simulink model "APVWith3DSimulation"  (R2022b)
settings: Solver=ode23tb  StartTime=0.0  StopTime=inf  MaxStep=1e-2  MinStep=1e-3  RelTol=1e-2
PreLoadFcn:
  | helperSLCreateUtilityBus(1);
StopFcn:
  | clear helperSLVisualizePath;
values from neighbouring files (symbols this model uses):
  costmap = vehicleCostmap(costmapStruct.Costs,          'FreeThreshold',     costmapStruct.FreeThreshold,          'OccupiedThreshold', costmapStruct.OccupiedThreshold,          'MapLocation',       costmapStruct.MapExtent([1, 3]),          'CellSize',          costmapStruct.CellSize,          'CollisionChecker',  ccConfig)    [helperSLVisualizePath.m]
undefined symbols (not defined in the file or in its folder): centerToRear, routePlan, startPose
libraries: drivinglib x2, drivingvehiclecontroller x2, simulink x2, simulink_extras x2, sim3dlib x1, sim3dautolib x1, autolibshared x1
CloseFcn:
  | clear plannerConfigBus ...
  | speedConfigBus ...
  | vehicleInfoBus ...
  | startPose ...
  | costmap ...
  | routeData ...
  | routePlan;
settings Model: Creator=The MathWorks, Inc.  LastModifiedBy=The MathWorks, Inc.
settings SolverCC: MaxConsecutiveMinStep=2  ZeroCrossAlgorithm=Adaptive  AlgebraicLoopSolver=TrustRegion  DecoupledContinuousIntegration=on  MinimalZcImpactIntegration=on
settings DataIOCC: SaveOutput=off  SignalLogging=off  DSMLogging=off  SaveTime=off  ReturnWorkspaceOutputs=off
settings DebuggingCC: UnconnectedInputMsg=warning  UnconnectedOutputMsg=warning  UnconnectedLineMsg=warning  PregeneratedLibrarySubsystemCodeDiagnostic=none  SFMachineParentedDataDiag=warning  ArithmeticOperatorsInVariantConditions=warning
settings ModelReferenceCC: EnableRefExpFcnMdlSchedulingChecks=on
settings SFSimCC: SimUseLocalCustomCode=off
settings RTWCC: RTWUseLocalCustomCode=off  DLArmComputeVersion=19.05

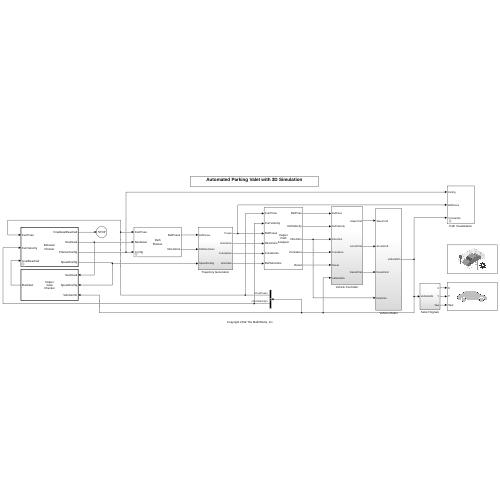
[thumbnail: Simulink's stored preview of the top-level diagram]
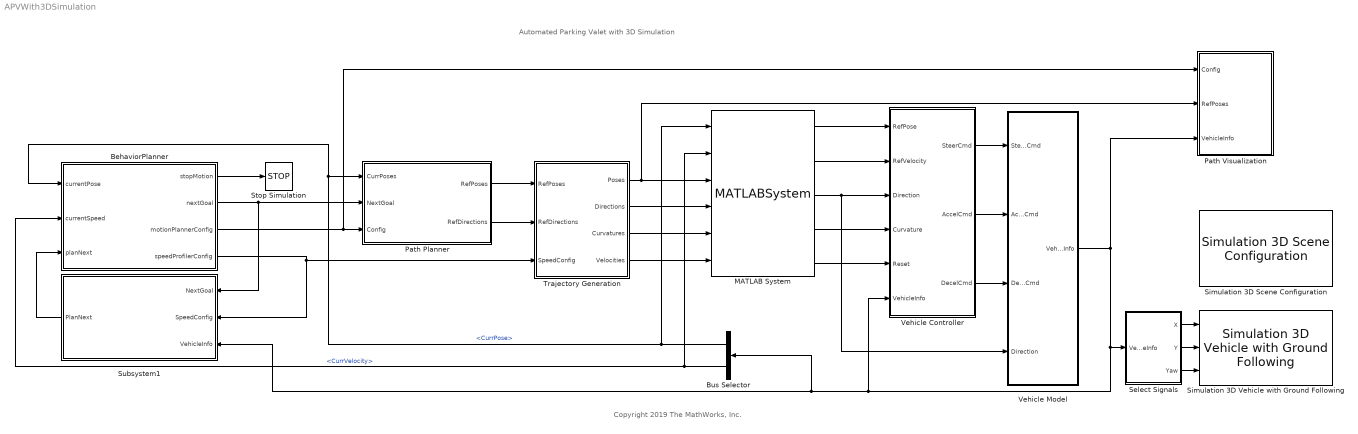
== system APVWith3DSimulation ==
  note: Copyright 2019 The MathWorks, Inc.
  note: Automated Parking Valet with 3D Simulation
  BehaviorPlanner : MATLAB Function  TreatAsAtomicUnit=on  mask{Costmap=costmap, RoutePlan=routePlan, StartSpeed=0}
      mask prompts: Costmap "Vehicle costmap:"; RoutePlan "Route plan:"; StartSpeed "Initial vehicle speed  [m/s]:"
      mask init:
      | validateattributes(Costmap, {'vehicleCostmap'}, {'scalar'});
      | validateattributes(RoutePlan, {'table'}, {'ncols', 3});
      | validateattributes(StartSpeed, {'double'}, {'scalar','nonnegative'})
      | 
      | routePlanStruct   = table2struct(RoutePlan);
      | startPose         = routePlanStruct(1).StartPose;
      | 
      | varagout          = helperSLCreateUtilityStruct(Costmap);
      | vehicleDimsStruct = varagout{1};
      | costmapStruct     = varagout{2};
  Bus Selector : BusSelector  OutputSignals=CurrPose,CurrVelocity
  MATLAB System : MATLABSystem  System=HelperPathAnalyzer  Wheelbase=2.6  HasResetOutput=on  SimulateUsing=Interpreted execution
      mask Type: HelperPathAnalyzer
      mask Display:
      | disp(['Helper' char(10) 'Path' char(10) 'Analyzer']);
      | port_label('input',1,'CurrPose');
      | port_label('input',2,'CurrVelocity');
      | port_label('input',3,'RefPoses');
      | port_label('input',4,'Directions');
      | port_label('input',5,'Curvatures');
      | port_label('input',6,'RefVelocities');
      | port_label('output',1,'RefPose');
      | port_label('output',2,'RefVelocity');
      | port_label('output',3,'Direction');
      | port_label('output',4,'Curvature');
      | port_label('output',5,'Reset');
  Path Planner : Subsystem  mask{Costmap=costmap, ParkCostmapSize=30}
      mask prompts: Costmap "Global vehicle costmap:"; ParkCostmapSize "Local vehicle costmap size (m):"
      mask init:
      | varagout = helperSLCreateUtilityStruct(Costmap);
      | vehicleDimsStruct = varagout{1};
      | costmapStruct     = varagout{2};
      mask DialogControl DescGroupVar Prompt: Path Planner Helper
      mask Display:
      | disp(['Path' char(10) 'Planner']);
      | port_label('input',1,'CurrPose');
      | port_label('input',2,'NextGoal');
      | port_label('input',3,'Config');
      | port_label('output',1,'RefPoses');
      | port_label('output',2,'Directions');
  Path Visualization : Subsystem  mask{Costmap=costmap, ParkCostmapSize=30}
      mask prompts: Costmap "Global vehicle costmap:"; ParkCostmapSize "Local vehicle costmap size (m):"
      mask init:
      | validateattributes(Costmap, {'vehicleCostmap'}, {'scalar'});
      | 
      | varagout          = helperSLCreateUtilityStruct(Costmap);
      | vehicleDimsStruct = varagout{1};
      | costmapStruct     = varagout{2};
      mask DialogControl DescTextVar Prompt: Visualize simulation results.
  Select Signals : Subsystem
  Simulation 3D Scene Configuration : sim3dlib/Simulation 3D Scene Configuration  Priority=0  ProjectFormat=Default Scenes  SceneDesc=Large parking lot  ProjectName=/mathworks/devel/bat/filer/batfs2510-0/BR2022bd.2041392.BR2022bd.2041231.pass/build/matlab/toolbox/shared/sim3d_projects/automotive_project/UE4/LinuxNoEditor/AutoVrtlEnv.sh  ScenePath=/Game/Maps/HwStrght  EnableOpenDRIVE=off  vehTagList={'Scene Origin';'SimulinkVehicle1'}  vehTag=SimulinkVehicle1  OpVisEn=off  Ts=1/40  EnableWindow=on  EnableRemoteAccess=off  EnableWeather=off  SunAltitude=40.0  SunAzimuth=90  clouds=10  wind=1  fog=0  rain=0  EnableGeospatial=off  OriginHeight=200  OriginLatitude=40.744652  OriginLongitude=-73.988864  MapStyle=Aerial  AdditionalAssetIDs=[]  UseAdvancedSunSky=off  SolarTime=11  TimeZone=-5  Day=21  Month=9  Year=2022  UseDaylightSavingTime=on  DSTStartDay=10  DSTStartMonth=3  DSTEndDay=3  DSTEndMonth=11  DSTSwitchHour=2  sensorTag=MainCamera3  sensorId=3  sensorName=MainCamera3  mountLoc=Origin  offsetFlag=off  tmountOffset=[0, 0, 0]  rmountOffset=[0, 0, 0]  HorizontalResolution=1280  VerticalResolution=720  HorizontalFOV=60  mountPoint=[0 0 0]  mountOrientation=[0 0 0]  aMode=3  ID=3  GeoTrigger=Inactive
  Simulation 3D Vehicle with Ground Following : sim3dautolib/Simulation 3D Vehicle with Ground Following  Priority=-1  PassVehMesh=Hatchback  MeshPath=/MathWorksSimulation/Vehicles/Muscle/Meshes/SK_MuscleCar.SK_MuscleCar  TrackWidth=1.9  WheelBase=3  WheelRadius=0.35  VehColor=Red  InitialPos=[startPose(1)+cosd(startPose(3))*centerToRear, startPose(2)+sind(startPose(3))*centerToRear, 0]  InitialRot=[0, 0, startPose(3)]  ActorName=SimulinkVehicle1  SampleTime=-1  ActorType=SimulinkVehicle  ID=1  aMode=3  ActorTag=SimulinkVehicle1  CoordinateScheme=ISO  VehLightsControl=off  HeadlightColor=[ 1, 1, 1 ]  HighBeamIntensity=100000  LowBeamIntensity=60000  HighBeamConeAngle=70  LowBeamConeAngle=70  LeftHeadlightOrientation=[ 0, 0 ]  RightHeadlightOrientation=[ 0, 0 ]  BrakelightIntensity=500  ReverselightIntensity=500  SignallightIntensity=500  SignallightPeriod=1  SignalPulseWidth=50  TransformOutportEnabled=off
  Stop Simulation : Stop
  Subsystem1 : Subsystem  TreatAsAtomicUnit=on  SystemSampleTime=0.1
      settings: MinAlgLoopOccurrences=on
      mask Display:
      | disp(['Helper' char(10) 'Goal' char(10) 'Checker']);
      | port_label('input',1,'NextGoal');
      | port_label('input',2,'SpeedConfig');
      | port_label('input',3,'VehicleInfo');
      | 
      | port_label('output',1,'PlanNext');
  Trajectory Generation : Subsystem
  Vehicle Controller : Subsystem
  Vehicle Model : Subsystem
  wires:
  BehaviorPlanner/2(nextGoal) -> Path Planner/2(NextGoal), Subsystem1/1(NextGoal)
  BehaviorPlanner/1(stopMotion) -> Stop Simulation/1
  BehaviorPlanner/4(speedProfilerConfig) -> Subsystem1/2(SpeedConfig), Trajectory Generation/3(SpeedConfig)
  Trajectory Generation/2(Directions) -> MATLAB System/4
  Trajectory Generation/1(Poses) -> Path Visualization/2(RefPoses), MATLAB System/3
  Subsystem1/1(PlanNext) -> BehaviorPlanner/3(planNext)
  MATLAB System/3 -> Vehicle Controller/3(Direction), Vehicle Model/4(Direction)
  Trajectory Generation/3(Curvatures) -> MATLAB System/5
  MATLAB System/2 -> Vehicle Controller/2(RefVelocity)
  MATLAB System/1 -> Vehicle Controller/1(RefPose)
  MATLAB System/4 -> Vehicle Controller/4(Curvature)
  Bus Selector/1 -> MATLAB System/1, BehaviorPlanner/1(currentPose), Path Planner/1(CurrPoses)  "<CurrPose>"
  Bus Selector/2 -> BehaviorPlanner/2(currentSpeed), MATLAB System/2  "<CurrVelocity>"
  MATLAB System/5 -> Vehicle Controller/5(Reset)
  Vehicle Controller/3(DecelCmd) -> Vehicle Model/3(DecelCmd)
  Vehicle Controller/1(SteerCmd) -> Vehicle Model/1(SteerCmd)
  Vehicle Controller/2(AccelCmd) -> Vehicle Model/2(AccelCmd)
  BehaviorPlanner/3(motionPlannerConfig) -> Path Visualization/1(Config), Path Planner/3(Config)
  Path Planner/1(RefPoses) -> Trajectory Generation/1(RefPoses)
  Path Planner/2(RefDirections) -> Trajectory Generation/2(RefDirections)
  Vehicle Model/1(VehicleInfo) -> Path Visualization/3(VehicleInfo), Vehicle Controller/6(VehicleInfo), Bus Selector/1, Subsystem1/3(VehicleInfo), Select Signals/1(VehicleInfo)
  Select Signals/1(X) -> Simulation 3D Vehicle with Ground Following/1
  Select Signals/2(Y) -> Simulation 3D Vehicle with Ground Following/2
  Select Signals/3(Yaw) -> Simulation 3D Vehicle with Ground Following/3
  Trajectory Generation/4(Velocities) -> MATLAB System/6

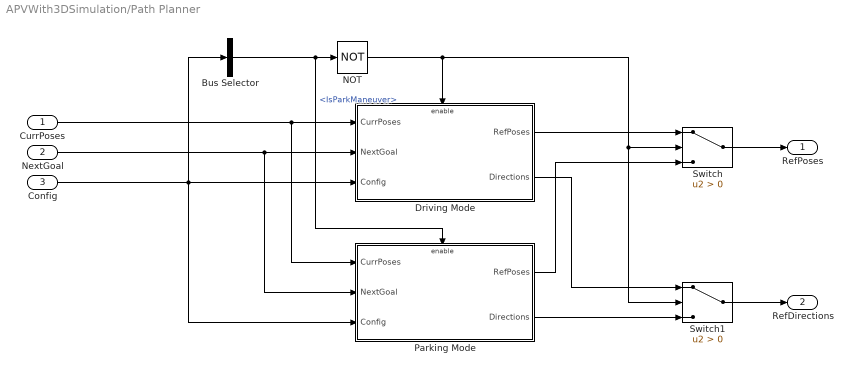
== system APVWith3DSimulation/Path Planner ==
  CurrPoses : Inport
  NextGoal : Inport  Port=2
  Config : Inport  Port=3
  Bus Selector : BusSelector  OutputSignals=IsParkManeuver
  Driving Mode : Subsystem
  NOT : Logic  Operator=NOT  IconShape=distinctive  AllPortsSameDT=off  OutDataTypeStr=boolean
  Parking Mode : Subsystem
  Switch : Switch  Criteria=u2 > Threshold  AllowDiffInputSizes=on  SaturateOnIntegerOverflow=off  InputSameDT=off
  Switch1 : Switch  Criteria=u2 > Threshold  AllowDiffInputSizes=on  SaturateOnIntegerOverflow=off  InputSameDT=off
  RefPoses : Outport  VectorParamsAs1DForOutWhenUnconnected=off
  RefDirections : Outport  Port=2  VectorParamsAs1DForOutWhenUnconnected=off
  wires:
  CurrPoses/1 -> Parking Mode/1(CurrPoses), Driving Mode/1(CurrPoses)
  NextGoal/1 -> Driving Mode/2(NextGoal), Parking Mode/2(NextGoal)
  Config/1 -> Bus Selector/1, Driving Mode/3(Config), Parking Mode/3(Config)
  Switch/1 -> RefPoses/1
  Switch1/1 -> RefDirections/1
  Driving Mode/1(RefPoses) -> Switch/1
  Parking Mode/1(RefPoses) -> Switch/3
  Driving Mode/2(Directions) -> Switch1/1
  Parking Mode/2(Directions) -> Switch1/3
  NOT/1 -> Driving Mode/Enable, Switch1/2, Switch/2
  Bus Selector/1 -> Parking Mode/Enable, NOT/1  "<IsParkManeuver>"

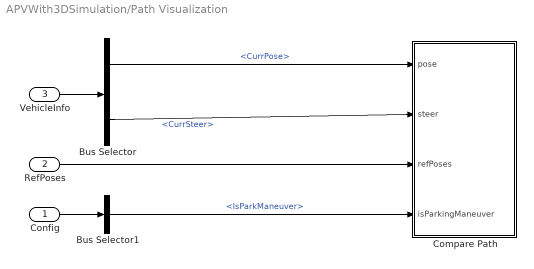
== system APVWith3DSimulation/Path Visualization ==
  Config : Inport
  RefPoses : Inport  Port=2
  VehicleInfo : Inport  Port=3
  Bus Selector : BusSelector  OutputSignals=CurrPose,CurrSteer
  Bus Selector1 : BusSelector  OutputSignals=IsParkManeuver
  Compare Path : MATLAB Function  TreatAsAtomicUnit=on
  wires:
  RefPoses/1 -> Compare Path/3(refPoses)
  VehicleInfo/1 -> Bus Selector/1
  Bus Selector/1 -> Compare Path/1(pose)  "<CurrPose>"
  Bus Selector/2 -> Compare Path/2(steer)  "<CurrSteer>"
  Config/1 -> Bus Selector1/1
  Bus Selector1/1 -> Compare Path/4(isParkingManeuver)  "<IsParkManeuver>"

== system APVWith3DSimulation/Select Signals ==
  VehicleInfo : Inport
  Bus Selector3 : BusSelector  OutputSignals=CurrPoseCenter
  Demux : Demux  Outputs=3
  X : Outport  VectorParamsAs1DForOutWhenUnconnected=off
  Y : Outport  Port=2  VectorParamsAs1DForOutWhenUnconnected=off
  Yaw : Outport  Port=3  VectorParamsAs1DForOutWhenUnconnected=off
  wires:
  Bus Selector3/1 -> Demux/1  "<CurrPoseCenter>"
  Demux/1 -> X/1
  VehicleInfo/1 -> Bus Selector3/1
  Demux/2 -> Y/1
  Demux/3 -> Yaw/1

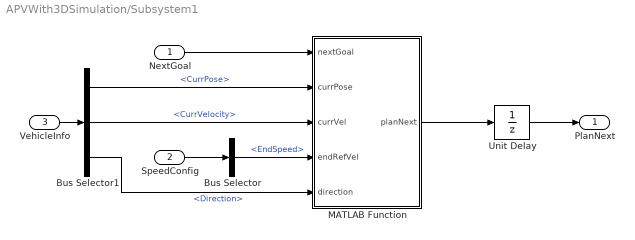
== system APVWith3DSimulation/Subsystem1 ==
  NextGoal : Inport
  SpeedConfig : Inport  Port=2
  VehicleInfo : Inport  Port=3
  Bus Selector : BusSelector  OutputSignals=EndSpeed
  Bus Selector1 : BusSelector  OutputSignals=CurrPose,CurrVelocity,Direction
  MATLAB Function : MATLAB Function  TreatAsAtomicUnit=on
  Unit Delay : UnitDelay  SampleTime=-1  HasFrameUpgradeWarning=on
  PlanNext : Outport  VectorParamsAs1DForOutWhenUnconnected=off
  wires:
  NextGoal/1 -> MATLAB Function/1(nextGoal)
  Bus Selector1/2 -> MATLAB Function/3(currVel)  "<CurrVelocity>"
  MATLAB Function/1(planNext) -> Unit Delay/1
  SpeedConfig/1 -> Bus Selector/1
  Unit Delay/1 -> PlanNext/1
  Bus Selector/1 -> MATLAB Function/4(endRefVel)  "<EndSpeed>"
  Bus Selector1/3 -> MATLAB Function/5(direction)  "<Direction>"
  VehicleInfo/1 -> Bus Selector1/1
  Bus Selector1/1 -> MATLAB Function/2(currPose)  "<CurrPose>"

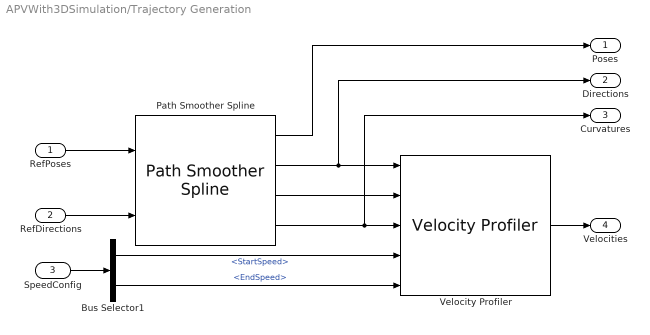
== system APVWith3DSimulation/Trajectory Generation ==
  RefPoses : Inport
  RefDirections : Inport  Port=2
  SpeedConfig : Inport  Port=3
  Bus Selector1 : BusSelector  OutputSignals=StartSpeed,EndSpeed
  Path Smoother Spline : drivinglib/Path Smoother Spline  NumSmoothPoses=500  MinSeparation=1e-3  SampleTime=-1  ShowOptionalOutports=on  SimulateUsing=Interpreted execution
  Velocity Profiler : drivinglib/Velocity Profiler  MaxLongitudinalAccel=2  MaxLongitudinalDecel=4  MaxSpeed=10  MaxLongitudinalJerk=1  MaxLateralAccel=2  ShowOptionalOutport=off  SampleTime=-1  SimulateUsing=Interpreted execution
  Poses : Outport  VectorParamsAs1DForOutWhenUnconnected=off
  Directions : Outport  Port=2  VectorParamsAs1DForOutWhenUnconnected=off
  Curvatures : Outport  Port=3  VectorParamsAs1DForOutWhenUnconnected=off
  Velocities : Outport  Port=4  VectorParamsAs1DForOutWhenUnconnected=off
  wires:
  Velocity Profiler/1 -> Velocities/1
  Path Smoother Spline/2 -> Directions/1, Velocity Profiler/1
  Path Smoother Spline/4 -> Curvatures/1, Velocity Profiler/3
  Bus Selector1/2 -> Velocity Profiler/5  "<EndSpeed>"
  RefPoses/1 -> Path Smoother Spline/1
  SpeedConfig/1 -> Bus Selector1/1
  Bus Selector1/1 -> Velocity Profiler/4  "<StartSpeed>"
  Path Smoother Spline/3 -> Velocity Profiler/2
  RefDirections/1 -> Path Smoother Spline/2
  Path Smoother Spline/1 -> Poses/1

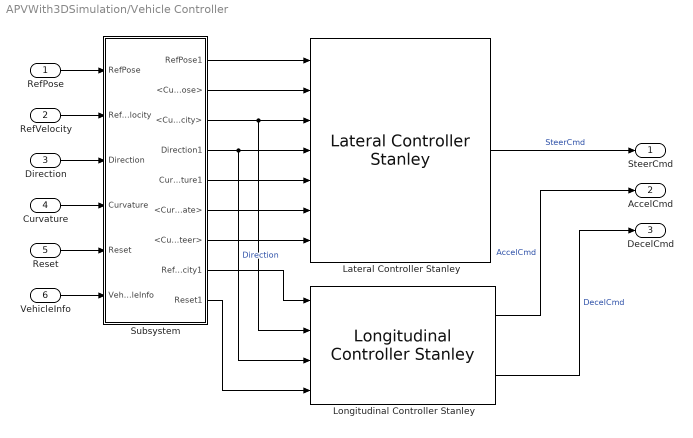
== system APVWith3DSimulation/Vehicle Controller ==
  RefPose : Inport  OutDataTypeStr=double  PortDimensions=[1 3]  SampleTime=[0.050000000000000003,0]
  RefVelocity : Inport  Port=2  OutDataTypeStr=double  PortDimensions=[1 1]  SampleTime=[0.050000000000000003,0]
  Direction : Inport  Port=3  OutDataTypeStr=double  PortDimensions=[1 1]  SampleTime=[0.050000000000000003,0]
  Curvature : Inport  Port=4  OutDataTypeStr=double  PortDimensions=[1 1]  SampleTime=[0.050000000000000003,0]
  Reset : Inport  Port=5  OutDataTypeStr=double  PortDimensions=[1 1]  SampleTime=[0.050000000000000003,0]
  VehicleInfo : Inport  Port=6  OutDataTypeStr=Bus: vehicleInfoBus
  Lateral Controller Stanley : drivingvehiclecontroller/Lateral Controller Stanley  ModelType=Dynamic bicycle model  PositionGainF=2  PositionGainR=2.5  YawRateGain=0.25  DelayGain=0.2  VehicleMass=1575  Lf=1.104  Lr=1.343  TireStiffness=19000  Wheelbase=2.8  MaxSteeringAngle=35
  Longitudinal Controller Stanley : drivingvehiclecontroller/Longitudinal Controller Stanley  Kp=2.5  Ki=1  SampleTime=0.05  MaxAcceleration=3  MaxDeceleration=6
  Subsystem : Subsystem
  SteerCmd : Outport  VectorParamsAs1DForOutWhenUnconnected=off
  AccelCmd : Outport  Port=2  VectorParamsAs1DForOutWhenUnconnected=off
  DecelCmd : Outport  Port=3  VectorParamsAs1DForOutWhenUnconnected=off
  wires:
  RefPose/1 -> Subsystem/1(RefPose)
  Subsystem/3(<CurrVelocity>) -> Lateral Controller Stanley/3, Longitudinal Controller Stanley/2
  Longitudinal Controller Stanley/1 -> AccelCmd/1  "AccelCmd"
  Subsystem/9(Reset1) -> Longitudinal Controller Stanley/4
  VehicleInfo/1 -> Subsystem/6(VehicleInfo)
  RefVelocity/1 -> Subsystem/2(RefVelocity)
  Longitudinal Controller Stanley/2 -> DecelCmd/1  "DecelCmd"
  Direction/1 -> Subsystem/3(Direction)
  Subsystem/4(Direction1) -> Lateral Controller Stanley/4, Longitudinal Controller Stanley/3  "Direction"
  Subsystem/2(<CurrPose>) -> Lateral Controller Stanley/2
  Reset/1 -> Subsystem/5(Reset)
  Subsystem/8(RefVelocity1) -> Longitudinal Controller Stanley/1
  Subsystem/1(RefPose1) -> Lateral Controller Stanley/1
  Lateral Controller Stanley/1 -> SteerCmd/1  "SteerCmd"
  Curvature/1 -> Subsystem/4(Curvature)
  Subsystem/6(<CurrYawRate>) -> Lateral Controller Stanley/6
  Subsystem/5(Curvature1) -> Lateral Controller Stanley/5
  Subsystem/7(<CurrSteer>) -> Lateral Controller Stanley/7

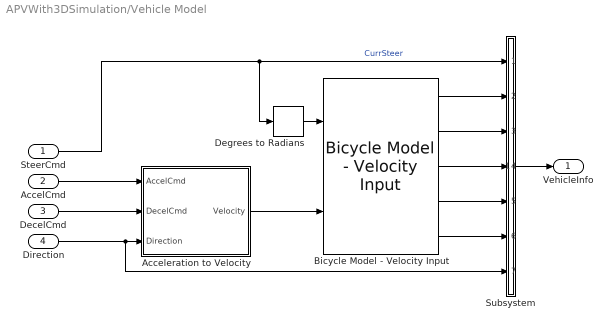
== system APVWith3DSimulation/Vehicle Model ==
  SteerCmd : Inport
  AccelCmd : Inport  Port=2
  DecelCmd : Inport  Port=3
  Direction : Inport  Port=4
  Acceleration to Velocity : Subsystem  TreatAsAtomicUnit=on
  Bicycle Model - Velocity Input : autolibshared/Bicycle Model - Velocity Input  trackMode=Single (bicycle)  inputMode=External longitudinal forces  frontSteerMode=on  rearSteerMode=off  windMode=off  muMode=off  extFMode=off  extMMode=off  aMode=3  NF=2  NR=2  m=1575  a=centerToFront  b=centerToRear  h=0.227  X_o=startPose(1)+cosd(startPose(3))*centerToRear  xdot_o=0  CalphaMode=off  sigmaMode=on  w=[1.4,1.4]  Cy_f=19e3  Cy_r=20e3  sigma_f=.1  sigma_r=.1  alpha_f_brk=[-.1 .1]  Cy_f_data=[-9e3 9e3]  alpha_r_brk=[-.1 .1]  Cy_r_data=[-9e3 9e3]  Y_o=startPose(2) +sind(startPose(3))*centerToRear  ydot_o=0  Izz=4000  psi_o=deg2rad(startPose(3))  r_o=0  Af=2  Cd=.3  Cl=.1  Cpm=.1  beta_w=[0:0.01:0.3]  Cs=[0:0.03:0.9]  Cym=[0:0.01:0.3]  Pabs=101325  Tair=273  g=9.81  mu=1  xdot_tol=.01  Fznom=5000  Fxtire_sat=1e6  Fytire_sat=1e6  longOff=0  latOff=0  vertOff=0
  Degrees to Radians : simulink_extras/Transformations/Degrees to Radians
  Subsystem : Subsystem
  VehicleInfo : Outport  VectorParamsAs1DForOutWhenUnconnected=off
  wires:
  Acceleration to Velocity/1(Velocity) -> Bicycle Model - Velocity Input/2
  Direction/1 -> Subsystem/7(<Direction>), Acceleration to Velocity/3(Direction)
  Degrees to Radians/1 -> Bicycle Model - Velocity Input/1
  SteerCmd/1 -> Degrees to Radians/1, Subsystem/1(CurrSteer)  "CurrSteer"
  DecelCmd/1 -> Acceleration to Velocity/2(DecelCmd)
  AccelCmd/1 -> Acceleration to Velocity/1(AccelCmd)
  Subsystem/1(VehicleInfo) -> VehicleInfo/1
  Bicycle Model - Velocity Input/1 -> Subsystem/2(Info)
  Bicycle Model - Velocity Input/2 -> Subsystem/3(xdot)
  Bicycle Model - Velocity Input/3 -> Subsystem/4(ydot)
  Bicycle Model - Velocity Input/4 -> Subsystem/5(psi)
  Bicycle Model - Velocity Input/5 -> Subsystem/6(r)

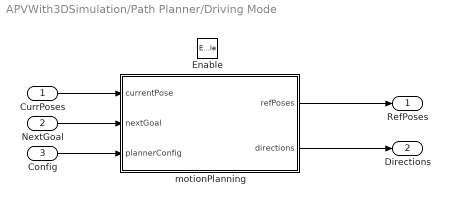
== system APVWith3DSimulation/Path Planner/Driving Mode ==
  CurrPoses : Inport
  NextGoal : Inport  Port=2
  Config : Inport  Port=3
  Enable : EnablePort  PropagateVarSize=During execution
  motionPlanning : MATLAB Function  TreatAsAtomicUnit=on
  RefPoses : Outport  VectorParamsAs1DForOutWhenUnconnected=off
  Directions : Outport  Port=2  VectorParamsAs1DForOutWhenUnconnected=off
  wires:
  motionPlanning/2(directions) -> Directions/1
  NextGoal/1 -> motionPlanning/2(nextGoal)
  Config/1 -> motionPlanning/3(plannerConfig)
  CurrPoses/1 -> motionPlanning/1(currentPose)
  motionPlanning/1(refPoses) -> RefPoses/1

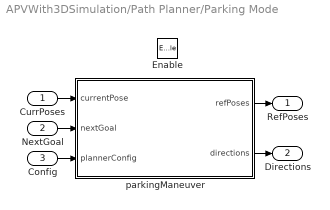
== system APVWith3DSimulation/Path Planner/Parking Mode ==
  CurrPoses : Inport
  NextGoal : Inport  Port=2
  Config : Inport  Port=3
  Enable : EnablePort  PropagateVarSize=During execution
  parkingManeuver : MATLAB Function  TreatAsAtomicUnit=on
  RefPoses : Outport  VectorParamsAs1DForOutWhenUnconnected=off
  Directions : Outport  Port=2  VectorParamsAs1DForOutWhenUnconnected=off
  wires:
  Config/1 -> parkingManeuver/3(plannerConfig)
  NextGoal/1 -> parkingManeuver/2(nextGoal)
  CurrPoses/1 -> parkingManeuver/1(currentPose)
  parkingManeuver/1(refPoses) -> RefPoses/1
  parkingManeuver/2(directions) -> Directions/1

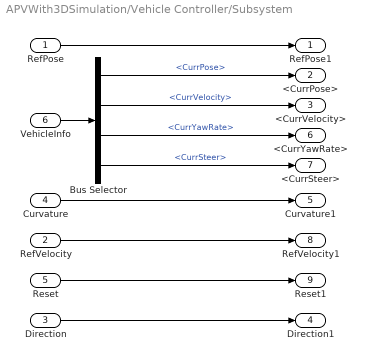
== system APVWith3DSimulation/Vehicle Controller/Subsystem ==
  RefPose : Inport
  RefVelocity : Inport  Port=2
  Direction : Inport  Port=3
  Curvature : Inport  Port=4
  Reset : Inport  Port=5
  VehicleInfo : Inport  Port=6
  Bus Selector : BusSelector  OutputSignals=CurrPose,CurrVelocity,CurrYawRate,CurrSteer
  RefPose1 : Outport  VectorParamsAs1DForOutWhenUnconnected=off
  <CurrPose> : Outport  Port=2  VectorParamsAs1DForOutWhenUnconnected=off
  <CurrVelocity> : Outport  Port=3  VectorParamsAs1DForOutWhenUnconnected=off
  Direction1 : Outport  Port=4  VectorParamsAs1DForOutWhenUnconnected=off
  Curvature1 : Outport  Port=5  VectorParamsAs1DForOutWhenUnconnected=off
  <CurrYawRate> : Outport  Port=6  VectorParamsAs1DForOutWhenUnconnected=off
  <CurrSteer> : Outport  Port=7  VectorParamsAs1DForOutWhenUnconnected=off
  RefVelocity1 : Outport  Port=8  VectorParamsAs1DForOutWhenUnconnected=off
  Reset1 : Outport  Port=9  VectorParamsAs1DForOutWhenUnconnected=off
  wires:
  Bus Selector/4 -> <CurrSteer>/1  "<CurrSteer>"
  Curvature/1 -> Curvature1/1
  Bus Selector/3 -> <CurrYawRate>/1  "<CurrYawRate>"
  Reset/1 -> Reset1/1
  RefPose/1 -> RefPose1/1
  Bus Selector/1 -> <CurrPose>/1  "<CurrPose>"
  Bus Selector/2 -> <CurrVelocity>/1  "<CurrVelocity>"
  RefVelocity/1 -> RefVelocity1/1
  VehicleInfo/1 -> Bus Selector/1
  Direction/1 -> Direction1/1

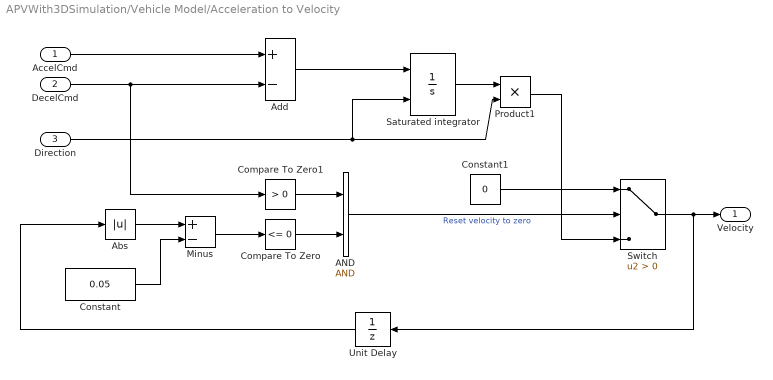
== system APVWith3DSimulation/Vehicle Model/Acceleration to Velocity ==
  AccelCmd : Inport  PortDimensions=[1 1]
  DecelCmd : Inport  Port=2  PortDimensions=[1 1]
  Direction : Inport  Port=3
  AND : Logic  IconShape=distinctive  AllPortsSameDT=off  OutDataTypeStr=boolean
  Abs : Abs  SaturateOnIntegerOverflow=off
  Add : Sum  Inputs=+-
  Compare To Zero : simulink/Logic and Bit Operations/Compare To Zero  relop=<=  OutDataTypeStr=boolean
  Compare To Zero1 : simulink/Logic and Bit Operations/Compare To Zero  relop=>  OutDataTypeStr=boolean
  Constant : Constant  Value=0.05
  Constant1 : Constant  Value=0
  Minus : Sum  Inputs=+-
  Product1 : Product
  Saturated integrator : Integrator  ExternalReset=either  LimitOutput=on  LowerSaturationLimit=0  AbsoluteTolerance=1e-3  ZeroCross=off
  Switch : Switch  Criteria=u2 > Threshold  SaturateOnIntegerOverflow=off  InputSameDT=off
  Unit Delay : UnitDelay  SampleTime=-1  HasFrameUpgradeWarning=on
  Velocity : Outport  VectorParamsAs1DForOutWhenUnconnected=off
  wires:
  Direction/1 -> Product1/2, Saturated integrator/2
  AccelCmd/1 -> Add/1
  Add/1 -> Saturated integrator/1
  DecelCmd/1 -> Compare To Zero1/1, Add/2
  Unit Delay/1 -> Abs/1
  Abs/1 -> Minus/1
  Constant/1 -> Minus/2
  Minus/1 -> Compare To Zero/1
  Compare To Zero/1 -> AND/2
  Compare To Zero1/1 -> AND/1
  AND/1 -> Switch/2  "Reset velocity to zero"
  Switch/1 -> Unit Delay/1, Velocity/1
  Constant1/1 -> Switch/1
  Saturated integrator/1 -> Product1/1
  Product1/1 -> Switch/3

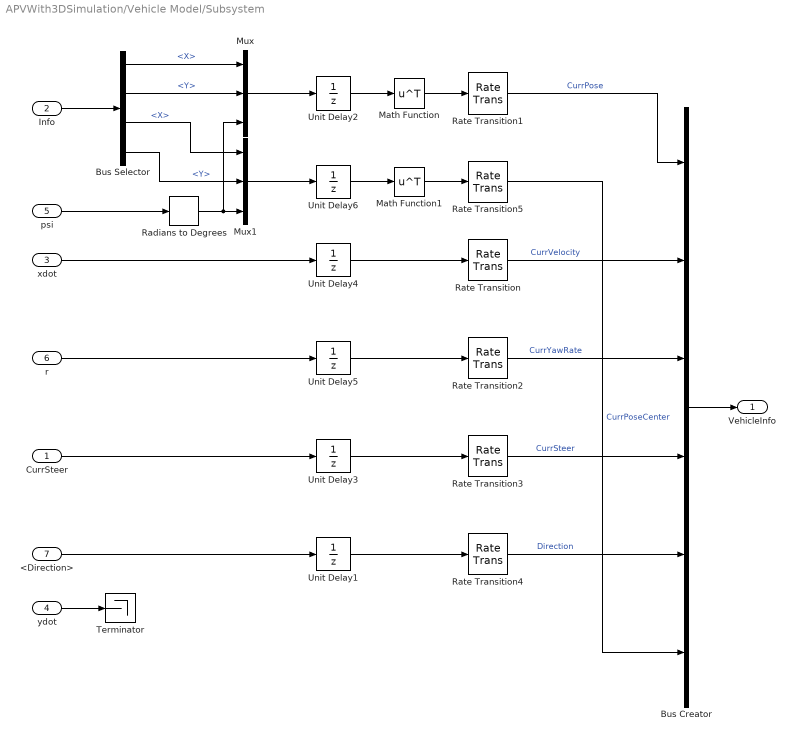
== system APVWith3DSimulation/Vehicle Model/Subsystem ==
  CurrSteer : Inport
  Info : Inport  Port=2
  xdot : Inport  Port=3
  ydot : Inport  Port=4
  psi : Inport  Port=5
  r : Inport  Port=6
  <Direction> : Inport  Port=7
  Bus Creator : BusCreator  Inputs=6  OutDataTypeStr=Bus: vehicleInfoBus  NonVirtualBus=on
  Bus Selector : BusSelector  OutputSignals=InertFrm.RearAxl.Disp.X,InertFrm.RearAxl.Disp.Y,InertFrm.Cg.Disp.X,InertFrm.Cg.Disp.Y
  Math Function : Math  Operator=transpose  SignedPower=on
  Math Function1 : Math  Operator=transpose  SignedPower=on
  Mux : Mux  Inputs=3
  Mux1 : Mux  Inputs=3
  Radians to Degrees : simulink_extras/Transformations/Radians to Degrees
  Rate Transition : RateTransition  OutPortSampleTime=0.05
  Rate Transition1 : RateTransition  InitialCondition=startPose  OutPortSampleTime=0.05
  Rate Transition2 : RateTransition  OutPortSampleTime=0.05
  Rate Transition3 : RateTransition  OutPortSampleTime=0.05
  Rate Transition4 : RateTransition  InitialCondition=1  OutPortSampleTime=0.05
  Rate Transition5 : RateTransition  InitialCondition=[startPose(1)-cosd(startPose(3))*centerToRear,startPose(2)-sind(startPose(3))*centerToRear,startPose(3)]  OutPortSampleTime=0.05
  Terminator : Terminator
  Unit Delay1 : UnitDelay  InitialCondition=1  SampleTime=-1  HasFrameUpgradeWarning=on
  Unit Delay2 : UnitDelay  InitialCondition=startPose  SampleTime=-1  HasFrameUpgradeWarning=on
  Unit Delay3 : UnitDelay  SampleTime=-1  HasFrameUpgradeWarning=on
  Unit Delay4 : UnitDelay  SampleTime=-1  HasFrameUpgradeWarning=on
  Unit Delay5 : UnitDelay  SampleTime=-1  HasFrameUpgradeWarning=on
  Unit Delay6 : UnitDelay  InitialCondition=[startPose(1)-cosd(startPose(3))*centerToRear,startPose(2)-sind(startPose(3))*centerToRear,startPose(3)]  SampleTime=-1  HasFrameUpgradeWarning=on
  VehicleInfo : Outport  VectorParamsAs1DForOutWhenUnconnected=off
  wires:
  Unit Delay1/1 -> Rate Transition4/1
  CurrSteer/1 -> Unit Delay3/1
  Unit Delay5/1 -> Rate Transition2/1
  <Direction>/1 -> Unit Delay1/1
  Unit Delay4/1 -> Rate Transition/1
  Math Function/1 -> Rate Transition1/1
  Rate Transition/1 -> Bus Creator/2  "CurrVelocity"
  Unit Delay3/1 -> Rate Transition3/1
  Rate Transition3/1 -> Bus Creator/4  "CurrSteer"
  Rate Transition1/1 -> Bus Creator/1  "CurrPose"
  Rate Transition2/1 -> Bus Creator/3  "CurrYawRate"
  Rate Transition4/1 -> Bus Creator/5  "Direction"
  Unit Delay2/1 -> Math Function/1
  Info/1 -> Bus Selector/1
  Radians to Degrees/1 -> Mux1/3, Mux/3
  Bus Selector/2 -> Mux/2  "<Y>"
  Bus Selector/1 -> Mux/1  "<X>"
  Mux/1 -> Unit Delay2/1
  xdot/1 -> Unit Delay4/1
  ydot/1 -> Terminator/1
  r/1 -> Unit Delay5/1
  Bus Creator/1 -> VehicleInfo/1
  Bus Selector/4 -> Mux1/2  "<Y>"
  Mux1/1 -> Unit Delay6/1
  Unit Delay6/1 -> Math Function1/1
  Math Function1/1 -> Rate Transition5/1
  Rate Transition5/1 -> Bus Creator/6  "CurrPoseCenter"
  Bus Selector/3 -> Mux1/1  "<X>"
  psi/1 -> Radians to Degrees/1

== matlab function APVWith3DSimulation/Path Visualization/Compare Path ==
  settings: updateMethod=DISCRETE  sampleTime=0.2
  data: pose input size=[1 3]; steer input; refPoses input; costmapStruct parameter; vehicleDimsStruct parameter; isParkingManeuver input; ParkCostmapSize parameter
function visualizePath(pose, steer, refPoses, costmapStruct, vehicleDimsStruct, isParkingManeuver, ParkCostmapSize)

%visualizePath Display simulation results.

coder.extrinsic('helperSLVisualizePath');

helperSLVisualizePath(pose, steer, refPoses, costmapStruct, vehicleDimsStruct, isParkingManeuver, ParkCostmapSize)

== matlab function APVWith3DSimulation/Path Planner/Driving Mode/motionPlanning ==
  settings: updateMethod=DISCRETE  sampleTime=0.1
  data: refPoses output size=[50 3]; currentPose input size=[1 3]; nextGoal input size=[1 3]; plannerConfig input Bus: plannerConfigBus; costmapStruct parameter; vehicleDimsStruct parameter; directions output size=[50 1]
function [refPoses, directions] = motionPlanning(currentPose, nextGoal, ...
    plannerConfig, costmapStruct, vehicleDimsStruct)

% %motionPlanning plan a feasible path using pathPlannerRRT.

%#codegen

persistent nextGoalPose posesInternal directionsInternal motionPlanner costmap

% Initialize persistent variables
if isempty(nextGoalPose)
    nextGoalPose = [0 0 0];
end

if isempty(posesInternal)
    posesInternal = [0 0 0];
end

if isempty(directionsInternal)
    directionsInternal = 1;
end

% Create vehicleDimensions object
vehicleDims = vehicleDimensions( ...
    vehicleDimsStruct.Length, ...
    vehicleDimsStruct.Width, ...
    vehicleDimsStruct.Height, ...
    'Wheelbase',          vehicleDimsStruct.Wheelbase, ...
    'RearOverhang',       vehicleDimsStruct.RearOverhang, ...
    'WorldUnits',         char(vehicleDimsStruct.WorldUnits));
ccConfig = inflationCollisionChecker(vehicleDims, 4);

% Initialize vehicleCostmap object
if isempty(costmap)
    costmap = vehicleCostmap(costmapStruct.Costs, ...
        'FreeThreshold',      costmapStruct.FreeThreshold, ...
        'OccupiedThreshold',  costmapStruct.OccupiedThreshold, ...
        'MapLocation',        costmapStruct.MapExtent([1, 3]), ...
        'CellSize',           costmapStruct.CellSize, ...
        'CollisionChecker',   ccConfig);
end

% Create pathPlannerRRT object
if isempty(motionPlanner)
    motionPlanner = pathPlannerRRT(costmap, ...
        'ConnectionDistance', plannerConfig.ConnectionDistance, ...
        'MinIterations',      plannerConfig.MinIterations, ...
        'GoalTolerance',      plannerConfig.GoalTolerance, ...
        'MinTurningRadius',   plannerConfig.MinTurningRadius);
end

% Only plan the path if there is a new goal
if ~isequal(nextGoalPose, nextGoal)
    nextGoalPose  = nextGoal;
    vehiclePose   = currentPose;
    
    motionPlanner.ConnectionDistance = plannerConfig.ConnectionDistance;
    motionPlanner.MinIterations      = plannerConfig.MinIterations;
    motionPlanner.GoalTolerance      = plannerConfig.GoalTolerance;
    motionPlanner.MinTurningRadius   = plannerConfig.MinTurningRadius;
    
    while true
        refPath       = plan(motionPlanner, vehiclePose, nextGoalPose);
        if refPath.Length>0
            break
        end
    end
    [refPoses, directions] = interpolate(refPath);
    
    posesInternal          = refPoses;
    directionsInternal     = directions;
else
    refPoses   = posesInternal;
    directions = directionsInternal;
end

if isempty(refPoses)
    error('No feasible path can be found.')
end

end

== matlab function APVWith3DSimulation/Subsystem1/MATLAB Function ==
  data: nextGoal input size=[1 3]; planNext output size=[1 1]; currPose input size=[1 3]; currVel input size=[1 1]; endRefVel input size=[1 1]; direction input
function planNext = goalCheker(nextGoal, currPose, currVel, endRefVel, direction)

planNext = helperGoalChecker(nextGoal, currPose, currVel, endRefVel, direction);

== matlab function APVWith3DSimulation/Path Planner/Parking Mode/parkingManeuver ==
  settings: updateMethod=DISCRETE  sampleTime=0.1
  data: refPoses output size=[50 3]; currentPose input size=[1 3]; nextGoal input size=[1 3]; plannerConfig input Bus: plannerConfigBus; costmapStruct parameter; vehicleDimsStruct parameter; directions output size=[50 1]; ParkCostmapSize parameter
function [refPoses, directions] = parkingManeuver(currentPose, nextGoal, ...
    plannerConfig, costmapStruct, vehicleDimsStruct, ParkCostmapSize)

%parkingManeuver plan a feasible path using pathPlannerRRT for parking

%#codegen

coder.extrinsic('helperPlotLocalCostmap');

persistent nextGoalPose posesInternal directionsInternal parkPlanner parkCostmap

% Initialize persistent variables
if isempty(nextGoalPose)
    nextGoalPose = [0 0 0];
end

if isempty(posesInternal)
    posesInternal = [0 0 0];
end

if isempty(directionsInternal)
    directionsInternal = 1;
end

% Create vehicleDimensions object
vehicleDims = vehicleDimensions( ...
    vehicleDimsStruct.Length, ...
    vehicleDimsStruct.Width, ...
    vehicleDimsStruct.Height, ...
    'Wheelbase',          vehicleDimsStruct.Wheelbase, ...
    'RearOverhang',       vehicleDimsStruct.RearOverhang, ...
    'WorldUnits',         char(vehicleDimsStruct.WorldUnits));
ccConfig = inflationCollisionChecker(vehicleDims, 5);

% Initialize vehicleCostmap object

if isempty(parkCostmap)
    costmap = vehicleCostmap(costmapStruct.Costs, ...
        'FreeThreshold',      costmapStruct.FreeThreshold, ...
        'OccupiedThreshold',  costmapStruct.OccupiedThreshold, ...
        'MapLocation',        costmapStruct.MapExtent([1, 3]), ...
        'CellSize',           costmapStruct.CellSize, ...
        'CollisionChecker',   ccConfig);
    
    parkCostmap = helperCreateLocalCostmap(costmap, currentPose, nextGoal, ParkCostmapSize);
end

% Create pathPlannerRRT object
if isempty(parkPlanner)
    parkPlanner = pathPlannerRRT(parkCostmap, ...
        'ConnectionDistance', plannerConfig.ConnectionDistance, ...
        'MinIterations',      plannerConfig.MinIterations, ...
        'GoalTolerance',      plannerConfig.GoalTolerance, ...
        'MinTurningRadius',   plannerConfig.MinTurningRadius);
end

% Only plan the path if there is a new goal
if ~isequal(nextGoalPose, nextGoal)
    nextGoalPose  = nextGoal;
    vehiclePose   = currentPose;
    
    parkPlanner.ConnectionDistance = plannerConfig.ConnectionDistance;
    parkPlanner.MinIterations      = plannerConfig.MinIterations;
    parkPlanner.GoalTolerance      = plannerConfig.GoalTolerance;
    parkPlanner.MinTurningRadius   = plannerConfig.MinTurningRadius;
    
    while true
        refPath       = plan(parkPlanner, vehiclePose, nextGoalPose);
        if refPath.Length>0
            break
        end
    end
    [refPoses, directions] = interpolate(refPath);
    
    posesInternal          = refPoses;
    directionsInternal     = directions;
else
    refPoses   = posesInternal;
    directions = directionsInternal;
end

if isempty(refPoses)
    error('No feasible path can be found.')
end

end

== matlab function APVWith3DSimulation/BehaviorPlanner ==
  settings: updateMethod=DISCRETE  sampleTime=0.1
  data: stopMotion output; nextGoal output double size=[1 3]; motionPlannerConfig output Bus: plannerConfigBus; speedProfilerConfig output Bus: speedConfigBus; routePlanStruct parameter; currentPose input size=[1 3]; currentSpeed input size=[1 1]; planNext input size=[1 1]; startPose parameter size=[1 3]; StartSpeed parameter
function [stopMotion, nextGoal, motionPlannerConfig, speedProfilerConfig] = ...
    behaviorPlanning(routePlanStruct, currentPose, currentSpeed, planNext, ...
    startPose, StartSpeed)

%behaviorPlanning generate navigation tasks and configurations for the 
%   Motion Planner block and the Trajectory Generator block.

nextGoal     = coder.nullcopy(zeros(1, 3)); %#ok<*NASGU>
stopMotion   = coder.nullcopy(logical(0));  %#ok<*LOGL>

persistent behavioralPlanner
persistent nextGoalPose plannerConfig speedConfig
persistent pose speed

if isempty(behavioralPlanner)
    
    % Initialize pose and speed
    pose  = startPose;
    speed = StartSpeed;
    
    % Initialize planner
    steerLimit = 30;
    behavioralPlanner = HelperBehavioralPlanner(routePlanStruct, steerLimit);
    [nextGoalPose, plannerConfig, speedConfig] = requestManeuver( ...
        behavioralPlanner, pose, speed);
end

pose  = currentPose;
speed = currentSpeed;

disTol = 1;
% Plan a new path when reaching the goal
if planNext && ~reachedDestination(behavioralPlanner)
    [nextGoalPose, plannerConfig, speedConfig] = requestManeuver( ...
        behavioralPlanner, pose, speed);
end

% Stop motion when reaching the destination
stopMotion = planNext && reachedDestination(behavioralPlanner) && ...
    norm(pose(1:2) - nextGoalPose(1:2)) < disTol;
    
nextGoal            = nextGoalPose;
motionPlannerConfig = plannerConfig;
speedProfilerConfig = speedConfig;

end
